simulink model "VirtualContactAgent"  (Simulink 7.1)
settings: Solver=ode45  StartTime=0.0  StopTime=10.0  RelTol=1e-3
settings Model: Creator=suarezjl  LastModifiedBy=suarezjl

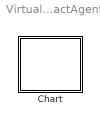
== system VirtualContactAgent ==
  Chart : Stateflow chart

== stateflow chart Chart ==
  state Averaging
    \\Octavia\\ISACControlBasisModule\VirtualContact\VirtualContact.AverageValues()
  state Stop
    \\Octavia\ISACControlBasisModule\VirtualContact\VirtualContact.Close()
  (default) -> Averaging : Start
  Averaging -> Stop [order 2] : Signal = "Stop"
  Averaging -> Averaging [order 1] : Default
